simulink model "pvt_tegs_vienna"  (R2023b)
settings: Solver=ode14x  StartTime=0.0  StopTime=3*24*3600  FixedStep=1  RelTol=1e-06
PreLoadFcn:
  | sscv_hybrid_solar_panel_data
values from neighbouring files (symbols this model uses):
  Inclination = struct()    [meteo_data_struct.m]
  Irradiance_si = struct()    [meteo_data_struct.m]
  Irradiance_ts = struct()    [meteo_data_struct.m]
  load = struct()    [pvt_tegs_data.m]
  month = months{m}    [AUTOMATICO_mix.m]    (also in AUTOMATICO_parallel.m; AUTOMATICO_series.m)
  panel = struct()    [pvt_tegs_data.m]
  pipe = struct()    [pvt_tegs_data.m]
  pumps = struct()    [pvt_tegs_data.m]
  T_ext = struct()    [meteo_data_struct.m]
  tank = struct()    [pvt_tegs_data.m]
  teg = struct()    [pvt_tegs_data.m]
libraries: fl_lib x69, nesl_utility x35, simulink x5, ee_lib x2, My_second_lib x1, SimscapeFluids_lib x1
(part 1 of 2)
CloseFcn:
  | try,close(figHandleSolarInputs),end
  | clear figHandleSolarInputs
  | try,close(figHandlePumpInputs),end
  | clear figHandlePumpInputs
  | try,close(figHandleOptics),end
  | clear figHandleOptics
  | try,close(figHandleOutputs),end
  | clear figHandleOutputs
Description:
  | Photovoltaic Thermal Hybrid Solar Panel.
  | %
settings Model: Creator=The MathWorks, Inc.  LastModifiedBy=Utente
settings SolverCC: MaxConsecutiveMinStep=10  MaxZcPerStep=1
settings DataIOCC: SaveOutput=off  SignalLogging=off  DSMLogging=off
settings OptimizationCC: ReuseModelBlockBuffer=off
settings DebuggingCC: UnconnectedInputMsg=warning  UnconnectedOutputMsg=warning  UnconnectedLineMsg=warning  ArithmeticOperatorsInVariantConditions=warning
settings ModelReferenceCC: EnableRefExpFcnMdlSchedulingChecks=on
settings SFSimCC: SimUseLocalCustomCode=off
settings RTWCC: RTWUseLocalCustomCode=off  DLArmComputeVersion=19.05
settings SimscapeCC: SimscapeLogType=all  SimscapeLogSimulationStatistics=on  SimscapeLogName=simlog_hybrid_solar_panel  SimscapeLogDataHistory=10000

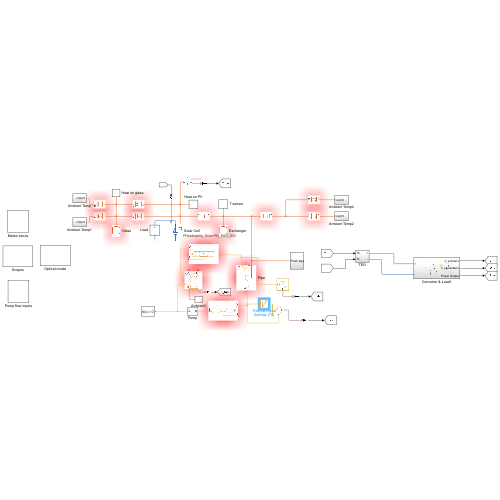
[thumbnail: Simulink's stored preview of the top-level diagram]
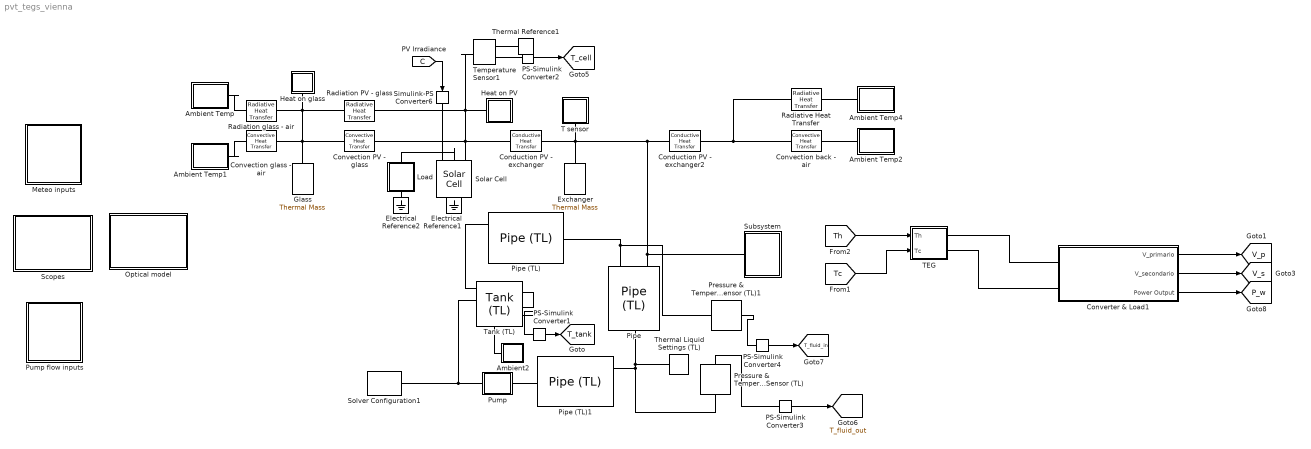
== system pvt_tegs_vienna ==
  Ambient Temp : Subsystem
  Ambient Temp1 : Subsystem
  Ambient Temp2 : Subsystem
  Ambient Temp4 : Subsystem
  Ambient2 : Subsystem
  Conduction PV - exchanger : fl_lib/Thermal/Thermal Elements/Conductive Heat Transfer  thermal_type=foundation.enum.ConstantVariableTabulated.Constant  wall_geometry=foundation.enum.ConductionWallGeometry.Planar  area=panel.geometry.Ncell*panel.geometry.Acell m^2  thickness=panel.heatTransfer.Le m  d_in=0.05 m  d_out=0.1 m  L=1 m  th_cond_min=10 W/(K*m)  th_cond=panel.heatTransfer.ke W/(m*K)  th_cond_TLU=[413, 401, 392, 383, 371, 357, 342] W/(K*m)  temp_TLU=[200, 273, 400, 600, 800, 1000, 1200] K  T_specify=off  T_priority=None  T=0 K  T_nominal_specify=off  T_nominal_unit=K  T_nominal_value=1  Q_specify=off  Q_priority=None  Q=0 W  Q_nominal_specify=off  Q_nominal_unit=W  Q_nominal_value=1
  Conduction PV - exchanger2 : fl_lib/Thermal/Thermal Elements/Conductive Heat Transfer  thermal_type=foundation.enum.ConstantVariableTabulated.Constant  wall_geometry=foundation.enum.ConductionWallGeometry.Planar  area=panel.geometry.Ncell*panel.geometry.Acell-teg.A_tot m^2  thickness=panel.heatTransfer.Le m  d_in=0.05 m  d_out=0.1 m  L=1 m  th_cond_min=10 W/(K*m)  th_cond=panel.heatTransfer.ke W/(m*K)  th_cond_TLU=[413, 401, 392, 383, 371, 357, 342] W/(K*m)  temp_TLU=[200, 273, 400, 600, 800, 1000, 1200] K  T_specify=off  T_priority=None  T=0 K  T_nominal_specify=off  T_nominal_unit=K  T_nominal_value=1  Q_specify=off  Q_priority=None  Q=0 W  Q_nominal_specify=off  Q_nominal_unit=W  Q_nominal_value=1
  Convection PV - glass : fl_lib/Thermal/Thermal Elements/Convective Heat Transfer  thermal_type=foundation.enum.constant_variable.constant  area=panel.geometry.Ncell*panel.geometry.Acell m^2  heat_tr_coeff=panel.heatTransfer.hgpv W/(m^2 * K)  min_heat_tr_coeff=1e-3 W/(K*m^2)  T_specify=off  T_priority=None  T=0 K  T_nominal_specify=off  T_nominal_unit=K  T_nominal_value=1  Q_specify=off  Q_priority=None  Q=0 W  Q_nominal_specify=off  Q_nominal_unit=W  Q_nominal_value=1
  Convection back - air : fl_lib/Thermal/Thermal Elements/Convective Heat Transfer  thermal_type=foundation.enum.constant_variable.constant  area=panel.geometry.Ncell*panel.geometry.Acell-teg.A_tot m^2  heat_tr_coeff=panel.heatTransfer.hba W/(m^2 * K)  min_heat_tr_coeff=1e-3 W/(K*m^2)  T_specify=off  T_priority=None  T=0 K  T_nominal_specify=off  T_nominal_unit=K  T_nominal_value=1  Q_specify=off  Q_priority=None  Q=0 W  Q_nominal_specify=off  Q_nominal_unit=W  Q_nominal_value=1
  Convection glass - air : fl_lib/Thermal/Thermal Elements/Convective Heat Transfer  thermal_type=foundation.enum.constant_variable.constant  area=panel.geometry.Ncell*panel.geometry.Acell m^2  heat_tr_coeff=panel.heatTransfer.hga W/(m^2 * K)  min_heat_tr_coeff=1e-3 W/(K*m^2)  T_specify=off  T_priority=None  T=0 K  T_nominal_specify=off  T_nominal_unit=K  T_nominal_value=1  Q_specify=off  Q_priority=None  Q=0 W  Q_nominal_specify=off  Q_nominal_unit=W  Q_nominal_value=1
  Converter & Load1 : Subsystem
  Electrical Reference1 : fl_lib/Electrical/Electrical Elements/Electrical Reference
  Electrical Reference2 : fl_lib/Electrical/Electrical Elements/Electrical Reference
  Exchanger : fl_lib/Thermal/Thermal Elements/Thermal Mass  mass_type=foundation.enum.constant_variable.constant  mass=panel.heatTransfer.Me kg  sp_heat=panel.heatTransfer.Ce J/kg/K  mass_min=1e-6 kg  num_ports=foundation.enum.numPorts2.one  m_specify=off  m_priority=High  m=1 kg  m_nominal_specify=off  m_nominal_unit=kg  m_nominal_value=1  T_specify=on  T_priority=High  T=panel.initial.Te0 K  T_nominal_specify=off  T_nominal_unit=K  T_nominal_value=1  Q_specify=off  Q_priority=None  Q=0 W  Q_nominal_specify=off  Q_nominal_unit=W  Q_nominal_value=1
  Glass : fl_lib/Thermal/Thermal Elements/Thermal Mass  mass_type=foundation.enum.constant_variable.constant  mass=panel.heatTransfer.Mg kg  sp_heat=panel.heatTransfer.Cg J/kg/K  mass_min=1e-6 kg  num_ports=foundation.enum.numPorts2.one  m_specify=off  m_priority=High  m=1 kg  m_nominal_specify=off  m_nominal_unit=kg  m_nominal_value=1  T_specify=on  T_priority=High  T=panel.initial.Tg0 K  T_nominal_specify=off  T_nominal_unit=K  T_nominal_value=1  Q_specify=off  Q_priority=None  Q=0 W  Q_nominal_specify=off  Q_nominal_unit=W  Q_nominal_value=1
  Heat on PV : Subsystem
  Heat on glass : Subsystem
  Load : Subsystem
  Meteo inputs : Subsystem
  Optical model : Subsystem
  PS-Simulink Converter1 : nesl_utility/PS-Simulink Converter  PhysicalDomain=network_engine_domain  SubClassName=ps_output  LeftPortType=input  RightPortType=output  PseudoPeriodic=off  Frequencies=[]  VectorFormat=inherit  Unit=inherit  AffineConversion=off
  PS-Simulink Converter2 : nesl_utility/PS-Simulink Converter  PhysicalDomain=network_engine_domain  SubClassName=ps_output  LeftPortType=input  RightPortType=output  PseudoPeriodic=off  Frequencies=[]  VectorFormat=inherit  Unit=K  AffineConversion=off
  PS-Simulink Converter3 : nesl_utility/PS-Simulink Converter  PhysicalDomain=network_engine_domain  SubClassName=ps_output  LeftPortType=input  RightPortType=output  PseudoPeriodic=off  Frequencies=[]  VectorFormat=inherit  Unit=inherit  AffineConversion=off
  PS-Simulink Converter4 : nesl_utility/PS-Simulink Converter  PhysicalDomain=network_engine_domain  SubClassName=ps_output  LeftPortType=input  RightPortType=output  PseudoPeriodic=off  Frequencies=[]  VectorFormat=inherit  Unit=inherit  AffineConversion=off
  Pipe : fl_lib/Thermal Liquid/Elements/Pipe (TL)  length=pipe.hx m  area=pipe.area m^2  Dh=pipe.Dh m  length_add=pipe.hx_eq_length m  roughness=pipe.roughness m  Re_lam=pipe.Re_lam  Re_tur=pipe.Re_tur  shape_factor=pipe.shape_factor  Nu_lam=pipe.Nu_lam  dynamic_compressibility=simscape.enum.onoff.off  inertia=simscape.enum.onoff.off  p0=0.101325 MPa  T0=Tm_month K  mdot0=0 kg/s
  Pipe (TL) : fl_lib/Thermal Liquid/Elements/Pipe (TL)  length=pipe.length m  area=pipe.area m^2  Dh=pipe.Dh m  length_add=pipe.eq_length1 m  roughness=pipe.roughness m  Re_lam=pipe.Re_lam  Re_tur=pipe.Re_tur  shape_factor=pipe.shape_factor  Nu_lam=pipe.Nu_lam  dynamic_compressibility=false  inertia=false  p0=0.101325 MPa  T0=Tm_month K  mdot0=0 kg/s
  Pipe (TL)1 : fl_lib/Thermal Liquid/Elements/Pipe (TL)  length=pipe.length m  area=pipe.area m^2  Dh=pipe.Dh m  length_add=pipe.eq_length2 m  roughness=pipe.roughness m  Re_lam=pipe.Re_lam  Re_tur=pipe.Re_tur  shape_factor=pipe.shape_factor  Nu_lam=pipe.Nu_lam  dynamic_compressibility=false  inertia=false  p0=0.101325 MPa  T0=Tm_month K  mdot0=0 kg/s
  Pressure & Temperature Sensor (TL) : fl_lib/Thermal Liquid/Sensors/Pressure & Temperature Sensor (TL)  reference=foundation.enum.MeasurementReference.absolute  pressure=false  pressure_spec=foundation.enum.PressureMeasementSpec.Absolute  temperature=true
      settings: InternalSimscapePortConfiguration="{\"Bottom\":[{\"id\":\"T\",\"label\":\"T\",\"type\":\"output\"}],\"Left\":[{\"id\":\"A\",\"label\":\"A\",\"type\":\"foundation.thermal_liquid.thermal_liquid\"}],\"Right\":[],\"Top\":[]}"
  Pressure & Temperature Sensor (TL)1 : fl_lib/Thermal Liquid/Sensors/Pressure & Temperature Sensor (TL)  reference=foundation.enum.MeasurementReference.absolute  pressure=false  pressure_spec=foundation.enum.PressureMeasementSpec.Absolute  temperature=true
      settings: InternalSimscapePortConfiguration="{\"Bottom\":[{\"id\":\"T\",\"label\":\"T\",\"type\":\"output\"}],\"Left\":[{\"id\":\"A\",\"label\":\"A\",\"type\":\"foundation.thermal_liquid.thermal_liquid\"}],\"Right\":[],\"Top\":[]}"
  Pump : Subsystem
  Pump flow inputs : Subsystem
  Radiation PV - glass : fl_lib/Thermal/Thermal Elements/Radiative Heat Transfer  area=panel.geometry.Ncell*panel.geometry.Acell m^2  rad_tr_coeff=5.670367e-8/(1/panel.heatTransfer.epsg + 1/panel.heatTransfer.epspv - 1) W/(m^2*K^4)  T_specify=off  T_priority=None  T=0 K  T_nominal_specify=off  T_nominal_unit=K  T_nominal_value=1  Q_specify=off  Q_priority=None  Q=0 W  Q_nominal_specify=off  Q_nominal_unit=W  Q_nominal_value=1
      settings: InternalSimscapePortConfiguration="{\"Bottom\":[],\"Left\":[{\"id\":\"A\",\"label\":\"A\",\"type\":\"foundation.thermal.thermal\"}],\"Right\":[{\"id\":\"B\",\"label\":\"B\",\"type\":\"foundation.thermal.thermal\"}],\"Top\":[]}"
  Radiation glass - air : fl_lib/Thermal/Thermal Elements/Radiative Heat Transfer  area=panel.geometry.Ncell*panel.geometry.Acell m^2  rad_tr_coeff=5.670367e-8*panel.heatTransfer.epsg W/(m^2*K^4)  T_specify=off  T_priority=None  T=0 K  T_nominal_specify=off  T_nominal_unit=K  T_nominal_value=1  Q_specify=off  Q_priority=None  Q=0 W  Q_nominal_specify=off  Q_nominal_unit=W  Q_nominal_value=1
      settings: InternalSimscapePortConfiguration="{\"Bottom\":[],\"Left\":[{\"id\":\"A\",\"label\":\"A\",\"type\":\"foundation.thermal.thermal\"}],\"Right\":[{\"id\":\"B\",\"label\":\"B\",\"type\":\"foundation.thermal.thermal\"}],\"Top\":[]}"
  Radiative Heat Transfer : fl_lib/Thermal/Thermal Elements/Radiative Heat Transfer  area=panel.geometry.Ncell*panel.geometry.Acell-teg.A_tot m^2  rad_tr_coeff=5.670367e-8/(1/pipe.emiss + 1/pipe.emiss_bricks - 1) W/(K^4*m^2)  T_specify=off  T_priority=None  T=0 K  T_nominal_specify=off  T_nominal_unit=K  T_nominal_value=1  Q_specify=off  Q_priority=None  Q=0 W  Q_nominal_specify=off  Q_nominal_unit=W  Q_nominal_value=1
      settings: InternalSimscapePortConfiguration="{\"Bottom\":[],\"Left\":[{\"id\":\"A\",\"label\":\"A\",\"type\":\"foundation.thermal.thermal\"}],\"Right\":[{\"id\":\"B\",\"label\":\"B\",\"type\":\"foundation.thermal.thermal\"}],\"Top\":[]}"
  Scopes : Subsystem
  Simulink-PS Converter6 : nesl_utility/Simulink-PS Converter  PhysicalDomain=network_engine_domain  SubClassName=ps_input  LeftPortType=input  RightPortType=output  PseudoPeriodic=off  Frequencies=[]  NoiseDistribution=none  NoiseParameters=[]  Unit=W/m^2  AffineConversion=off  FilteringAndDerivatives=provide  SimscapeFilterOrder=1  InputFilterTimeConstant=0.001  UdotUserProvided=0
  Solar Cell : ee_lib/Sources/Solar Cell  Tag={'toolbox/physmod/elec/library/m/ee_lib_parts';'Sources/Solar_Cell/Philadelphia_Solar/PS_M60_305.xml'}  prm=3  Isc=9.78 A  Voc=0.66918 V  Is=2.35776661208729e-07 A  Is2=1.71964843290271e-09 A  Iph=9.78001180187482 A  Ir0=1000 W/m^2  ec=1.48486924498379  N2=1.8278696613491  Rs=0.000864040468174528 Ohm  Rp=759.804445024526 Ohm  N_series=60  N_parallel=1  TIPH1=0.000600001676771431 1/K  EG=1.12 eV  TXIS1=5.6792037392937  TXIS2=14.7305501462979  TRS1=0.146242343009721  TRP1=0 % Parameter not set  Tmeas=25 degC  TFIXED=25 degC  thermal_mass=100 % Parameter not set J/K  initial_temperature=25 degC
      settings: AttributesFormatString=Philadelphia_Solar:PS_M60_305  InternalSimscapePortConfiguration="{\"Bottom\":[],\"Left\":[{\"id\":\"Ir\",\"label\":\"Ir\",\"type\":\"input\"},{\"id\":\"p\",\"label\":\"+\",\"type\":\"foundation.electrical.electrical\"},{\"id\":\"H\",\"label\":\"H\",\"type\":\"foundation.thermal.thermal\"}],\"Right\":[{\"id\":\"n\",\"label\":\"-\",\"type\":\"foundation.electrical.electrical\"}],\"Top\":[]}"
  Solver Configuration1 : nesl_utility/Solver Configuration  PhysicalDomain=network_engine_domain  SubClassName=solver  LeftPortType=input  RightPortType=generic  Tones=[]  Harmonics=[]  SimulateNoise=off  Profile=off  UseLocalSampling=off  EnableSwitchedLinearOptims=on  FrequencyDomain=off  UseCCode=off  RelTol=0.001  AbsTol=0.001  MinStep=1e-09  ToWorkspace=off  RevertToSquareIcSolve=off  NumHomotopyIterations=100  PhasorMode=off  PhasorModeNumHarmonics=1  ConsistencySolver=NEWTON_XTOL_AFTER_FTOL  IndexReductionMethod=DerivativeReplacement  DoDC=off  ResidualTolerance=1e-09  ConsistencyTolSource=GLOBAL  ConsistencyAbsTol=0.001  ConsistencyRelTol=0.001  ConsistencyTolFactor=0.001  UseLocalSolver=off  LocalSolverChoice=NE_BACKWARD_EULER_ADVANCER  ResolveIndetEquations=on  FunctionEvalNumThread=1  LocalSolverSampleTime=0.001  DoFixedCost=off  MaxNonlinIter=3  MaxModeIter=2  ComputeImpulses=off  ImpulseIterations=2  LinearAlgebra=auto  LinearAlgebraNumThread=0  EquationFormulation=NE_TIME_EF  DelaysMemoryBudget=1024  AutomaticFiltering=on  FilteringTimeConstant=0.001  PartitionStorageMethod=AS_NEEDED  PartitionMemoryBudget=1024  PartitionMethod=ROBUST  MultibodyUseLocalSolver=off  MultibodyLocalSolverChoice=ODE1  MultibodyLocalSolverSampleTime=0.001
  Subsystem : Subsystem
  T sensor : Subsystem
  TEG : Subsystem
  Tank (TL) : SimscapeFluids_lib/Thermal Liquid/Tanks & Accumulators/Tank (TL)  num_inlet=fluids.thermal_liquid.tanks_accumulators.enum.NumInlet.Two  pressure_spec=fluids.thermal_liquid.tanks_accumulators.enum.TankPressureSpec.Atmospheric  tank_pressure=0.101325 MPa  volume_spec=fluids.thermal_liquid.tanks_accumulators.enum.TankVolumeSpec.Constant  tank_area=tank.Atank m^2  level_TLU=[0, 3, 5] m  volume_TLU=[0, 4, 6] m^3  inlet_height_A=0.1 m  inlet_area_A=0.01 m^2  inlet_heights_AB=[0,0] m  inlet_areas_AB=[tank.Atank,tank.Atank] m^2  inlet_heights_ABC=[.1, .1, .1] m  inlet_areas_ABC=[.01, .01, .01] m^2  inlet_heights_ABCD=0.1 * ones(1, 4) m  inlet_areas_ABCD=0.01 * ones(1, 4) m^2  inlet_heights_ABCDE=0.1 * ones(1, 5) m  inlet_areas_ABCDE=0.01 * ones(1, 5) m^2  inlet_heights_ABCDEF=0.1 * ones(1, 6) m  inlet_areas_ABCDEF=0.01 * ones(1, 6) m^2  level_check=simscape.enum.assert.action.error  capacity_check=simscape.enum.assert.action.warn  max_capacity=tank.Volmax m^3  g=9.81 m/s^2  level_specify=on  level_priority=Low  level=tank.Voltank0/tank.Atank m  level_nominal_specify=off  level_nominal_unit=m  level_nominal_value=1  volume_specify=on  volume_priority=High  volume=tank.Voltank0 m^3  volume_nominal_specify=off  volume_nominal_unit=m^3  volume_nominal_value=1  mass_specify=off  mass_priority=None  mass=5000 kg  mass_nominal_specify=off  mass_nominal_unit=kg  mass_nominal_value=1  T_I_specify=on  T_I_priority=High  T_I=Tm_month K  T_I_nominal_specify=off  T_I_nominal_unit=K  T_I_nominal_value=1
      settings: InternalSimscapePortConfiguration="{\"Bottom\":[{\"id\":\"H\",\"label\":\"H\",\"type\":\"foundation.thermal.thermal\"},{\"id\":\"T_out\",\"label\":\"T\",\"type\":\"output\"}],\"Left\":[{\"id\":\"A\",\"label\":\"A\",\"type\":\"foundation.thermal_liquid.thermal_liquid\"},{\"id\":\"B\",\"label\":\"B\",\"type\":\"foundation.thermal_liquid.thermal_liquid\"}],\"Right\":[],\"Top\":[{\"id\":\"V_out\",\"label\":\"V\",\"type\":\"output\"},{\"id\":\"L_out\",\"label\":\"L\",\"type\":\"output\"}]}"
  Temperature Sensor1 : fl_lib/Thermal/Thermal Sensors/Temperature Sensor  temperature_measure=foundation.enum.MeasurementReference.difference
  Thermal Liquid Settings (TL) : fl_lib/Thermal Liquid/Utilities/Thermal Liquid Settings (TL)  table_dimensions=foundation.enum.table_dimensions_TL.one_dimensional  T_TLU=[263.16, 273.16:20:373.16]' K  p_TLU=[0.01, 0.1, 5 : 5 : 50] MPa  p_atm=0.101325 MPa  pT_region_flag=foundation.enum.pT_region_TL.min_max  T_min=273.16 K  T_max=363.16 K  p_min=0.05 MPa  p_max=50 MPa  T_min_1D=263.16 K  T_max_1D=373.16 K  p_min_1D=0.05 MPa  p_max_1D=50 MPa  pT_validity_TLU=[1, 1, 1, 1, 1, 1, 1, 1, 1, 1, 1, 1; 1, 1, 1, 1, 1, 1, 1, 1, 1, 1, 1, 1; 1, 1, 1, 1, 1, 1, 1, 1, 1, 1, 1, 1; 1, 1, 1, 1, 1, 1, 1, 1, 1, 1, 1, 1; 1, 1, 1, 1, 1, 1, 1, 1, 1, 1, 1, 1; 0, 1, 1, 1, 1, 1, 1, 1, 1, 1, 1, 1; 0, 1, 1, 1, 1, 1, 1, 1, 1, 1, 1, 1; 0, 1, 1, 1, 1, 1, 1, 1, 1, 1, 1, 1; 0, 1, 1, 1, 1, 1, 1, 1, 1, 1, 1, 1; 0, 1, 1, 1, 1, 1, 1, 1, 1, 1, 1, 1; 0, 0, 1, 1, 1, 1, 1, 1, 1, 1, 1, 1]  properties_range_check=simscape.enum.assert.action.error  rho_parameterization_2D=foundation.enum.rho_parameterization_2D.rho_beta_alpha  rho_parameterization_1D=foundation.enum.rho_parameterization_1D.rho_vector  rho_TLU=[999.7973, 999.8431, 1002.3216, 1004.8218, 1007.293, 1009.7358, 1012.1506, 1014.5379, 1016.8979, 1019.2311, 1021.538, 1023.8188; 999.6579, 999.7009, 1002.0303, 1004.382, 1006.7084, 1009.0101, 1011.2874, 1013.5407, 1015.7703, 1017.9766, 1020.1599, 1022.3206; 998.1632, 998.2045, 1000.4375, 1002.6924, 1004.9239, 1007.1324, 1009.3183, 1011.4819, 1013.6236, 1015.7438, 1017.8428, 1019.921; 995.6057, 995.6458, 997.81864, 1000.0128, 1002.1841, 1004.3332, 1006.4603, 1008.566, 1010.6505, 1012.7144, 1014.758, 1016.7815; 992.1724, 992.2119, 994.35133, 996.5113, 998.6484, 1000.7633, 1002.8563, 1004.928, 1006.9788, 1009.009, 1011.0192, 1013.0097; 988.02, 988.0299, 990.15684, 992.3035, 994.4268, 996.5273, 998.6056, 1000.6622, 1002.6976, 1004.7123, 1006.7067, 1008.6813; 983.18, 983.1901, 985.3217, 987.4721, 989.5983, 991.7008, 993.7803, 995.8374, 997.8726, 999.8864, 1001.8795, 1003.8522; 977.75, 977.7583, 979.9094, 982.0783, 984.2216, 986.34, 988.4343, 990.505, 992.5529, 994.5786, 996.5825, 998.5654; 971.77, 971.7836, 973.96734, 976.1678, 978.3409, 980.4876, 982.6087, 984.7049, 986.7768, 988.8254, 990.8511, 992.8545; 965.26, 965.3023, 967.53107, 969.7753, 971.9901, 974.1764, 976.3354, 978.4676, 980.5741, 982.6556, 984.7129, 986.7465; 958.62, 958.6315, 960.627, 962.9267, 965.1944, 967.4314, 969.6387, 971.8173, 973.9681, 976.0921, 978.19, 980.2628] kg/m^3  beta_TLU=[1.9649, 1.9654, 1.9929, 2.0213, 2.0499, 2.0787, 2.1078, 2.1372, 2.1668, 2.1966, 2.2268, 2.2572; 2.0913, 2.0918, 2.1191, 2.1471, 2.1752, 2.2036, 2.2322, 2.261, 2.2899, 2.3191, 2.3485, 2.3781; 2.1786, 2.1791, 2.2067, 2.235, 2.2634, 2.2919, 2.3206, 2.3494, 2.3784, 2.4075, 2.4367, 2.4661; 2.2332, 2.2337, 2.2619, 2.2908, 2.3197, 2.3487, 2.3778, 2.407, 2.4363, 2.4657, 2.4951, 2.5246; 2.26, 2.2605, 2.2895, 2.3191, 2.3487, 2.3784, 2.4081, 2.4378, 2.4675, 2.4973, 2.5272, 2.5571; 2.2638, 2.2638, 2.2936, 2.324, 2.3544, 2.3848, 2.4151, 2.4455, 2.4758, 2.5062, 2.5365, 2.5669; 2.2472, 2.2472, 2.2779, 2.3092, 2.3403, 2.3715, 2.4025, 2.4336, 2.4646, 2.4955, 2.5264, 2.5573; 2.214, 2.214, 2.2455, 2.2776, 2.3096, 2.3415, 2.3733, 2.405, 2.4367, 2.4683, 2.4998, 2.5313; 2.1668, 2.1668, 2.1992, 2.2321, 2.2649, 2.2976, 2.3301, 2.3626, 2.3949, 2.4272, 2.4593, 2.4914; 2.1081, 2.1081, 2.1413, 2.175, 2.2086, 2.2421, 2.2754, 2.3085, 2.3415, 2.3744, 2.4072, 2.4399; 2.0494, 2.0494, 2.0739, 2.1084, 2.1428, 2.177, 2.211, 2.2449, 2.2786, 2.3121, 2.3455, 2.3788] GPa  alpha_TLU=1e-4 * [-.679, -.676, -.49, -.307, -.13, .041, .206, .365, .519, .668, .811, .949; .878, .881, .998, 1.114, 1.227, 1.337, 1.445, 1.549, 1.651, 1.75, 1.846, 1.939; 2.068, 2.069, 2.141, 2.213, 2.283, 2.352, 2.42, 2.486, 2.551, 2.614, 2.676, 2.736; 3.034, 3.035, 3.074, 3.113, 3.152, 3.191, 3.229, 3.267, 3.305, 3.341, 3.377, 3.413; 3.855, 3.856, 3.87, 3.884, 3.899, 3.914, 3.93, 3.946, 3.961, 3.977, 3.993, 4.009; 4.578, 4.578, 4.572, 4.566, 4.562, 4.558, 4.555, 4.552, 4.55, 4.549, 4.548, 4.547; 5.233, 5.233, 5.209, 5.186, 5.165, 5.144, 5.125, 5.107, 5.09, 5.074, 5.059, 5.045; 5.84, 5.84, 5.801, 5.762, 5.725, 5.691, 5.657, 5.625, 5.595, 5.566, 5.538, 5.512; 6.414, 6.414, 6.36, 6.307, 6.256, 6.208, 6.161, 6.117, 6.074, 6.033, 5.994, 5.956; 6.967, 6.967, 6.898, 6.831, 6.766, 6.705, 6.646, 6.589, 6.535, 6.482, 6.432, 6.384; 7.519, 7.519, 7.423, 7.342, 7.264, 7.189, 7.118, 7.049, 6.983, 6.92, 6.859, 6.8] 1/K  rho_TLU_2=[999.7973, 999.8431, 1002.3216, 1004.8218, 1007.293, 1009.7358, 1012.1506, 1014.5379, 1016.8979, 1019.2311, 1021.538, 1023.8188; 999.6579, 999.7009, 1002.0303, 1004.382, 1006.7084, 1009.0101, 1011.2874, 1013.5407, 1015.7703, 1017.9766, 1020.1599, 1022.3206; 998.1632, 998.2045, 1000.4375, 1002.6924, 1004.9239, 1007.1324, 1009.3183, 1011.4819, 1013.6236, 1015.7438, 1017.8428, 1019.921; 995.6057, 995.6458, 997.81864, 1000.0128, 1002.1841, 1004.3332, 1006.4603, 1008.566, 1010.6505, 1012.7144, 1014.758, 1016.7815; 992.1724, 992.2119, 994.35133, 996.5113, 998.6484, 1000.7633, 1002.8563, 1004.928, 1006.9788, 1009.009, 1011.0192, 1013.0097; 988.02, 988.0299, 990.15684, 992.3035, 994.4268, 996.5273, 998.6056, 1000.6622, 1002.6976, 1004.7123, 1006.7067, 1008.6813; 983.18, 983.1901, 985.3217, 987.4721, 989.5983, 991.7008, 993.7803, 995.8374, 997.8726, 999.8864, 1001.8795, 1003.8522; 977.75, 977.7583, 979.9094, 982.0783, 984.2216, 986.34, 988.4343, 990.505, 992.5529, 994.5786, 996.5825, 998.5654; 971.77, 971.7836, 973.96734, 976.1678, 978.3409, 980.4876, 982.6087, 984.7049, 986.7768, 988.8254, 990.8511, 992.8545; 965.26, 965.3023, 967.53107, 969.7753, 971.9901, 974.1764, 976.3354, 978.4676, 980.5741, 982.6556, 984.7129, 986.7465; 958.62, 958.6315, 960.627, 962.9267, 965.1944, 967.4314, 969.6387, 971.8173, 973.9681, 976.0921, 978.19, 980.2628] kg/m^3  rho_ref_3=998.21 kg/m^3  T_ref_3=293.16 K  p_ref_3=0.101325 MPa  beta_const_3=2.1791 GPa  alpha_const_3=2.0691e-4 1/K  rho_TLU_4=[1038, 1036, 1030, 1022, 1014, 1006, 997]' kg/m^3  beta_const_4=3.4 GPa  p_ref_4=0.101325 MPa  rho_ref_5=998.21 kg/m^3  T_ref_5=293.16 K  p_ref_5=0.101325 MPa  beta_const_5=2.1791 GPa  alpha_const_5=2.0691e-4 1/K  u_parameterization_2D=foundation.enum.u_parameterization_2D.u_cp  u_parameterization_1D=foundation.enum.u_parameterization_1D.cp  u_TLU=[.0002, .0018, .086, .1588, .219, .267, .3034, .3288, .3436, .3483, .3435, .3294; 42.062, 42.06, 41.935, 41.804, 41.668, 41.527, 41.382, 41.233, 41.081, 40.924, 40.763, 40.599; 83.953, 83.948, 83.651, 83.349, 83.049, 82.749, 82.451, 82.153, 81.856, 81.56, 81.265, 80.971; 125.77, 125.76, 125.31, 124.86, 124.41, 123.97, 123.53, 123.1, 122.68, 122.25, 121.84, 121.42; 167.57, 167.56, 166.96, 166.37, 165.79, 165.21, 164.65, 164.09, 163.54, 163, 162.46, 161.94; 209.36, 209.36, 208.63, 207.9, 207.19, 206.48, 205.79, 205.11, 204.45, 203.79, 203.14, 202.5; 251.19, 251.19, 250.33, 249.47, 248.62, 247.79, 246.98, 246.18, 245.39, 244.62, 243.86, 243.12; 293.06, 293.06, 292.07, 291.07, 290.1, 289.14, 288.2, 287.28, 286.38, 285.49, 284.62, 283.77; 334.99, 334.99, 333.86, 332.73, 331.63, 330.54, 329.48, 328.44, 327.41, 326.41, 325.43, 324.46; 377, 377, 375.73, 374.46, 373.22, 372, 370.81, 369.64, 368.5, 367.38, 366.27, 365.19; 419.01, 419.01, 417.69, 416.27, 414.89, 413.54, 412.21, 410.91, 409.64, 408.4, 407.17, 405.98] kJ/kg  cp_TLU=[4.2199, 4.2194, 4.1957, 4.1726, 4.1508, 4.13, 4.1103, 4.0916, 4.0738, 4.0569, 4.0408, 4.0254; 4.1955, 4.1951, 4.1769, 4.1592, 4.1422, 4.1259, 4.1103, 4.0954, 4.0812, 4.0676, 4.0545, 4.0421; 4.1843, 4.184, 4.169, 4.1543, 4.1401, 4.1264, 4.1133, 4.1007, 4.0885, 4.0768, 4.0656, 4.0548; 4.1801, 4.1798, 4.1667, 4.1538, 4.1413, 4.1293, 4.1177, 4.1064, 4.0956, 4.0851, 4.075, 4.0653; 4.1796, 4.1794, 4.1675, 4.1558, 4.1444, 4.1334, 4.1227, 4.1123, 4.1023, 4.0926, 4.0832, 4.0741; 4.1813, 4.1813, 4.1702, 4.1592, 4.1484, 4.138, 4.1279, 4.1181, 4.1086, 4.0993, 4.0903, 4.0816; 4.185, 4.185, 4.1742, 4.1636, 4.1532, 4.1432, 4.1334, 4.1239, 4.1146, 4.1056, 4.0969, 4.0884; 4.1901, 4.1901, 4.1795, 4.169, 4.1588, 4.1489, 4.1393, 4.1299, 4.1207, 4.1118, 4.1032, 4.0947; 4.1968, 4.1968, 4.1862, 4.1757, 4.1655, 4.1555, 4.1458, 4.1364, 4.1273, 4.1183, 4.1096, 4.1012; 4.2052, 4.2052, 4.1944, 4.1837, 4.1733, 4.1632, 4.1534, 4.1438, 4.1345, 4.1255, 4.1166, 4.108; 4.2136, 4.2136, 4.2045, 4.1935, 4.1828, 4.1724, 4.1623, 4.1524, 4.1429, 4.1335, 4.1245, 4.1157] kJ/kg/K  u_TLU_2=[.0002, .0018, .086, .1588, .219, .267, .3034, .3288, .3436, .3483, .3435, .3294; 42.062, 42.06, 41.935, 41.804, 41.668, 41.527, 41.382, 41.233, 41.081, 40.924, 40.763, 40.599; 83.953, 83.948, 83.651, 83.349, 83.049, 82.749, 82.451, 82.153, 81.856, 81.56, 81.265, 80.971; 125.77, 125.76, 125.31, 124.86, 124.41, 123.97, 123.53, 123.1, 122.68, 122.25, 121.84, 121.42; 167.57, 167.56, 166.96, 166.37, 165.79, 165.21, 164.65, 164.09, 163.54, 163, 162.46, 161.94; 209.36, 209.36, 208.63, 207.9, 207.19, 206.48, 205.79, 205.11, 204.45, 203.79, 203.14, 202.5; 251.19, 251.19, 250.33, 249.47, 248.62, 247.79, 246.98, 246.18, 245.39, 244.62, 243.86, 243.12; 293.06, 293.06, 292.07, 291.07, 290.1, 289.14, 288.2, 287.28, 286.38, 285.49, 284.62, 283.77; 334.99, 334.99, 333.86, 332.73, 331.63, 330.54, 329.48, 328.44, 327.41, 326.41, 325.43, 324.46; 377, 377, 375.73, 374.46, 373.22, 372, 370.81, 369.64, 368.5, 367.38, 366.27, 365.19; 419.01, 419.01, 417.69, 416.27, 414.89, 413.54, 412.21, 410.91, 409.64, 408.4, 407.17, 405.98] kJ/kg  cp_TLU_3=[4.2199, 4.2194, 4.1957, 4.1726, 4.1508, 4.13, 4.1103, 4.0916, 4.0738, 4.0569, 4.0408, 4.0254; 4.1955, 4.1951, 4.1769, 4.1592, 4.1422, 4.1259, 4.1103, 4.0954, 4.0812, 4.0676, 4.0545, 4.0421; 4.1843, 4.184, 4.169, 4.1543, 4.1401, 4.1264, 4.1133, 4.1007, 4.0885, 4.0768, 4.0656, 4.0548; 4.1801, 4.1798, 4.1667, 4.1538, 4.1413, 4.1293, 4.1177, 4.1064, 4.0956, 4.0851, 4.075, 4.0653; 4.1796, 4.1794, 4.1675, 4.1558, 4.1444, 4.1334, 4.1227, 4.1123, 4.1023, 4.0926, 4.0832, 4.0741; 4.1813, 4.1813, 4.1702, 4.1592, 4.1484, 4.138, 4.1279, 4.1181, 4.1086, 4.0993, 4.0903, 4.0816; 4.185, 4.185, 4.1742, 4.1636, 4.1532, 4.1432, 4.1334, 4.1239, 4.1146, 4.1056, 4.0969, 4.0884; 4.1901, 4.1901, 4.1795, 4.169, 4.1588, 4.1489, 4.1393, 4.1299, 4.1207, 4.1118, 4.1032, 4.0947; 4.1968, 4.1968, 4.1862, 4.1757, 4.1655, 4.1555, 4.1458, 4.1364, 4.1273, 4.1183, 4.1096, 4.1012; 4.2052, 4.2052, 4.1944, 4.1837, 4.1733, 4.1632, 4.1534, 4.1438, 4.1345, 4.1255, 4.1166, 4.108; 4.2136, 4.2136, 4.2045, 4.1935, 4.1828, 4.1724, 4.1623, 4.1524, 4.1429, 4.1335, 4.1245, 4.1157] kJ/kg/K  u_TLU_4=[.0018; 42.06; 83.948; 125.76; 167.56; 209.36; 251.19; 293.06; 334.99; 377; 418.01] kJ/kg  cp_TLU_5=[3.85, 3.87, 3.90, 3.93, 3.96, 3.99, 4.02]' kJ/kg/K  nu_TLU=[1.7917, 1.7914, 1.7763, 1.7615, 1.7473, 1.7338, 1.7208, 1.7085, 1.6967, 1.6854, 1.6747, 1.6645; 1.3061, 1.3059, 1.2986, 1.2914, 1.2845, 1.2779, 1.2716, 1.2656, 1.2598, 1.2543, 1.2491, 1.2441; 1.0032, 1.0032, .9995, .9959, .9924, .9891, .9859, .9829, .9801, .9774, .9748, .9724; .8006, .8005, .7987, .797, .7953, .7937, .7922, .7908, .7894, .7881, .787, .7859; .6577, .6577, .657, .6562, .6555, .6548, .6543, .6537, .6532, .6528, .6523, .652; .553, .553, .5529, .5527, .5526, .5525, .5524, .5524, .5524, .5524, .5524, .5525; .4739, .4739, .4741, .4743, .4745, .4747, .475, .4753, .4755, .4758, .4762, .4765; .4127, .4127, .4131, .4135, .4139, .4143, .4148, .4152, .4157, .4162, .4167, .4172; .3643, .3643, .3648, .3654, .3659, .3665, .367, .3676, .3682, .3688, .3694, .37; .3254, .3254, .3261, .3267, .3273, .328, .3286, .3293, .3299, .3306, .3312, .3319; .2866, .2866, .2945, .2952, .2959, .2965, .2972, .2979, .2986, .2993, .3, .3007] mm^2/s  nu_TLU_2=[5, 3, 1.6, 1.0, 0.7, 0.52, 0.41]' mm^2/s  k_TLU=[561.04, 561.09, 563.8, 566.56, 569.32, 572.08, 574.82, 577.54, 580.24, 582.92, 585.57, 588.18; 580.02, 580.07, 582.45, 584.88, 587.32, 589.75, 592.18, 594.61, 597.02, 599.42, 601.8, 604.16; 598.44, 598.48, 600.73, 603.03, 605.33, 607.64, 609.94, 612.24, 614.54, 616.82, 619.1, 621.36; 615.48, 615.52, 617.73, 620, 622.26, 624.54, 626.81, 629.07, 631.34, 633.6, 635.85, 638.09; 630.6, 630.64, 632.87, 635.15, 637.44, 639.72, 642.01, 644.29, 646.57, 648.84, 651.11, 653.36; 643.61, 643.61, 645.88, 648.21, 650.53, 652.86, 655.18, 657.51, 659.82, 662.14, 664.44, 666.74; 654.39, 654.39, 656.73, 659.12, 661.5, 663.89, 666.27, 668.65, 671.02, 673.38, 675.74, 678.09; 663.13, 663.13, 665.54, 668, 670.46, 672.91, 675.36, 677.8, 680.24, 682.67, 685.09, 687.5; 670.02, 670.02, 672.51, 675.05, 677.59, 680.12, 682.64, 685.16, 687.67, 690.17, 692.66, 695.14; 675.27, 675.27, 677.85, 680.48, 683.11, 685.73, 688.34, 690.94, 693.53, 696.11, 698.68, 701.24; 680.52, 680.52, 681.77, 684.5, 687.22, 689.94, 692.64, 695.34, 698.02, 700.69, 703.35, 706] mW/m/K  k_TLU_2=[498, 500, 512, 521, 531, 540, 550]' mW/m/K
  Thermal Reference1 : fl_lib/Thermal/Thermal Elements/Thermal Reference
  tag scope: P_w=global, T_cell=global, T_fluid_in=global, T_fluid_out=global, T_tank=global, V_p=global, V_s=global
  wires:
  Converter & Load1/1(V_primario) -> [V_p]
  PS-Simulink Converter4/1 -> [T_fluid_in]
  Converter & Load1/3(Power Output) -> [P_w]
  Converter & Load1/2(V_secondario) -> [V_s]
  PS-Simulink Converter2/1 -> [T_cell]
  PS-Simulink Converter3/1 -> [T_fluid_out]
  [Tc] -> TEG/2(Tc)
  [C] -> Simulink-PS Converter6/1
  PS-Simulink Converter1/1 -> [T_tank]
  [Th] -> TEG/1(Th)
  connections:
  Pipe/LConn2 -- Subsystem/RConn1 -- Conduction PV - exchanger2/LConn1 -- Conduction PV - exchanger/RConn1 -- T sensor/LConn1 -- Exchanger/LConn1
  Pipe/RConn1 -- Thermal Liquid Settings (TL)/RConn1 -- Pressure & Temperature Sensor (TL)/LConn1 -- Pipe (TL)1/LConn1
  Pump/LConn1 -- Tank (TL)/LConn2 -- Solver Configuration1/RConn1
  Pipe/LConn1 -- Pipe (TL)/RConn1 -- Pressure & Temperature Sensor (TL)1/LConn1
  Radiation glass - air/LConn1 -- Convection glass - air/LConn1 -- Convection PV - glass/RConn1 -- Glass/LConn1 -- Radiation PV - glass/RConn1 -- Heat on glass/LConn1
  Convection back - air/LConn1 -- Radiative Heat Transfer/LConn1 -- Conduction PV - exchanger2/RConn1
  Convection PV - glass/LConn1 -- Radiation PV - glass/LConn1 -- Temperature Sensor1/LConn1 -- Heat on PV/LConn1 -- Conduction PV - exchanger/LConn1 -- Solar Cell/LConn3
  Thermal Reference1/LConn1 -- Temperature Sensor1/RConn1
  TEG/RConn2 -- Converter & Load1/LConn2
  Pressure & Temperature Sensor (TL)1/RConn1 -- PS-Simulink Converter4/LConn1
  Convection back - air/RConn1 -- Ambient Temp2/LConn1
  Temperature Sensor1/RConn2 -- PS-Simulink Converter2/LConn1
  Pipe (TL)1/RConn1 -- Pump/RConn1
  Solar Cell/RConn1 -- Electrical Reference1/LConn1
  PS-Simulink Converter3/LConn1 -- Pressure & Temperature Sensor (TL)/RConn1
  Ambient Temp4/LConn1 -- Radiative Heat Transfer/RConn1
  Ambient Temp/LConn1 -- Radiation glass - air/RConn1
  Solar Cell/LConn1 -- Simulink-PS Converter6/RConn1
  TEG/RConn1 -- Converter & Load1/LConn1
  Tank (TL)/RConn1 -- Ambient2/LConn1
  Ambient Temp1/LConn1 -- Convection glass - air/RConn1
  Tank (TL)/RConn2 -- PS-Simulink Converter1/LConn1
  Load/LConn1 -- Electrical Reference2/LConn1
  Pipe (TL)/LConn1 -- Tank (TL)/LConn1
  Solar Cell/LConn2 -- Load/RConn1

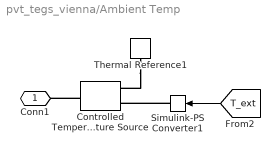
== system pvt_tegs_vienna/Ambient Temp ==
  Controlled Temperature Source : fl_lib/Thermal/Thermal Sources/Controlled Temperature Source
  Simulink-PS Converter1 : nesl_utility/Simulink-PS Converter  PhysicalDomain=network_engine_domain  SubClassName=ps_input  LeftPortType=input  RightPortType=output  PseudoPeriodic=off  Frequencies=[]  NoiseDistribution=none  NoiseParameters=[]  Unit=K  AffineConversion=off  FilteringAndDerivatives=provide  SimscapeFilterOrder=1  InputFilterTimeConstant=0.001  UdotUserProvided=0
  Thermal Reference1 : fl_lib/Thermal/Thermal Elements/Thermal Reference
  Conn1 : PMIOPort  Side=Left
  wires:
  [T_ext] -> Simulink-PS Converter1/1
  connections:
  Simulink-PS Converter1/RConn1 -- Controlled Temperature Source/RConn1
  Thermal Reference1/LConn1 -- Controlled Temperature Source/RConn2
  Controlled Temperature Source/LConn1 -- Conn1/RConn1

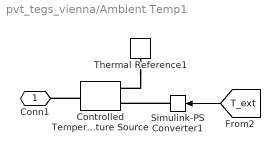
== system pvt_tegs_vienna/Ambient Temp1 ==
  Controlled Temperature Source : fl_lib/Thermal/Thermal Sources/Controlled Temperature Source
  Simulink-PS Converter1 : nesl_utility/Simulink-PS Converter  PhysicalDomain=network_engine_domain  SubClassName=ps_input  LeftPortType=input  RightPortType=output  PseudoPeriodic=off  Frequencies=[]  NoiseDistribution=none  NoiseParameters=[]  Unit=K  AffineConversion=off  FilteringAndDerivatives=provide  SimscapeFilterOrder=1  InputFilterTimeConstant=0.001  UdotUserProvided=0
  Thermal Reference1 : fl_lib/Thermal/Thermal Elements/Thermal Reference
  Conn1 : PMIOPort  Side=Left
  wires:
  [T_ext] -> Simulink-PS Converter1/1
  connections:
  Controlled Temperature Source/LConn1 -- Conn1/RConn1
  Thermal Reference1/LConn1 -- Controlled Temperature Source/RConn2
  Simulink-PS Converter1/RConn1 -- Controlled Temperature Source/RConn1

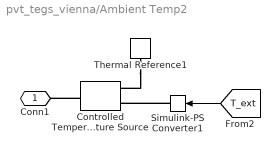
== system pvt_tegs_vienna/Ambient Temp2 ==
  Controlled Temperature Source : fl_lib/Thermal/Thermal Sources/Controlled Temperature Source
  Simulink-PS Converter1 : nesl_utility/Simulink-PS Converter  PhysicalDomain=network_engine_domain  SubClassName=ps_input  LeftPortType=input  RightPortType=output  PseudoPeriodic=off  Frequencies=[]  NoiseDistribution=none  NoiseParameters=[]  Unit=K  AffineConversion=off  FilteringAndDerivatives=provide  SimscapeFilterOrder=1  InputFilterTimeConstant=0.001  UdotUserProvided=0
  Thermal Reference1 : fl_lib/Thermal/Thermal Elements/Thermal Reference
  Conn1 : PMIOPort  Side=Left
  wires:
  [T_ext] -> Simulink-PS Converter1/1
  connections:
  Simulink-PS Converter1/RConn1 -- Controlled Temperature Source/RConn1
  Thermal Reference1/LConn1 -- Controlled Temperature Source/RConn2
  Controlled Temperature Source/LConn1 -- Conn1/RConn1

== system pvt_tegs_vienna/Ambient Temp4 ==
  Controlled Temperature Source : fl_lib/Thermal/Thermal Sources/Controlled Temperature Source
  Simulink-PS Converter1 : nesl_utility/Simulink-PS Converter  PhysicalDomain=network_engine_domain  SubClassName=ps_input  LeftPortType=input  RightPortType=output  PseudoPeriodic=off  Frequencies=[]  NoiseDistribution=none  NoiseParameters=[]  Unit=K  AffineConversion=off  FilteringAndDerivatives=provide  SimscapeFilterOrder=1  InputFilterTimeConstant=0.001  UdotUserProvided=0
  Thermal Reference1 : fl_lib/Thermal/Thermal Elements/Thermal Reference
  Conn1 : PMIOPort  Side=Left
  wires:
  [T_ext] -> Simulink-PS Converter1/1
  connections:
  Controlled Temperature Source/LConn1 -- Conn1/RConn1
  Thermal Reference1/LConn1 -- Controlled Temperature Source/RConn2
  Simulink-PS Converter1/RConn1 -- Controlled Temperature Source/RConn1

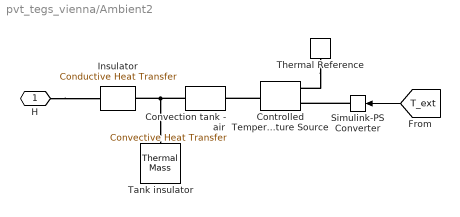
== system pvt_tegs_vienna/Ambient2 ==
  Controlled Temperature Source : fl_lib/Thermal/Thermal Sources/Controlled Temperature Source
  Convection tank - air : fl_lib/Thermal/Thermal Elements/Convective Heat Transfer  thermal_type=foundation.enum.constant_variable.constant  area=2*pi*sqrt(tank.Atank/pi)*tank.Volmax/tank.Atank+2*tank.Atank m^2  heat_tr_coeff=tank.hta W/(m^2 * K)  min_heat_tr_coeff=1e-3 W/(K*m^2)  T_specify=off  T_priority=None  T=0 K  T_nominal_specify=off  T_nominal_unit=K  T_nominal_value=1  Q_specify=off  Q_priority=None  Q=0 W  Q_nominal_specify=off  Q_nominal_unit=W  Q_nominal_value=1
  Insulator : fl_lib/Thermal/Thermal Elements/Conductive Heat Transfer  thermal_type=foundation.enum.ConstantVariableTabulated.Constant  wall_geometry=foundation.enum.ConductionWallGeometry.Planar  area=2*pi*sqrt(tank.Atank/pi)*tank.Volmax/tank.Atank+2*tank.Atank m^2  thickness=tank.Lins m  d_in=0.05 m  d_out=0.1 m  L=1 m  th_cond_min=10 W/(K*m)  th_cond=tank.kins W/(m*K)  th_cond_TLU=[413, 401, 392, 383, 371, 357, 342] W/(K*m)  temp_TLU=[200, 273, 400, 600, 800, 1000, 1200] K  T_specify=off  T_priority=None  T=0 K  T_nominal_specify=off  T_nominal_unit=K  T_nominal_value=1  Q_specify=off  Q_priority=None  Q=0 W  Q_nominal_specify=off  Q_nominal_unit=W  Q_nominal_value=1
  Simulink-PS Converter : nesl_utility/Simulink-PS Converter  PhysicalDomain=network_engine_domain  SubClassName=ps_input  LeftPortType=input  RightPortType=output  PseudoPeriodic=off  Frequencies=[]  NoiseDistribution=none  NoiseParameters=[]  Unit=K  AffineConversion=off  FilteringAndDerivatives=provide  SimscapeFilterOrder=1  InputFilterTimeConstant=0.001  UdotUserProvided=0
  Tank insulator : fl_lib/Thermal/Thermal Elements/Thermal Mass  mass_type=foundation.enum.constant_variable.constant  mass=tank.insul_mass kg  sp_heat=tank.spec_heat J/(K*kg)  mass_min=1e-6 kg  num_ports=foundation.enum.numPorts2.one  m_specify=off  m_priority=High  m=1 kg  m_nominal_specify=off  m_nominal_unit=kg  m_nominal_value=1  T_specify=off  T_priority=High  T=300 K  T_nominal_specify=off  T_nominal_unit=K  T_nominal_value=1  Q_specify=off  Q_priority=None  Q=0 W  Q_nominal_specify=off  Q_nominal_unit=W  Q_nominal_value=1
  Thermal Reference : fl_lib/Thermal/Thermal Elements/Thermal Reference
  H : PMIOPort  Side=Left
  wires:
  [T_ext] -> Simulink-PS Converter/1
  connections:
  H/RConn1 -- Insulator/LConn1
  Convection tank - air/LConn1 -- Insulator/RConn1 -- Tank insulator/LConn1
  Controlled Temperature Source/LConn1 -- Convection tank - air/RConn1
  Simulink-PS Converter/RConn1 -- Controlled Temperature Source/RConn1
  Thermal Reference/LConn1 -- Controlled Temperature Source/RConn2

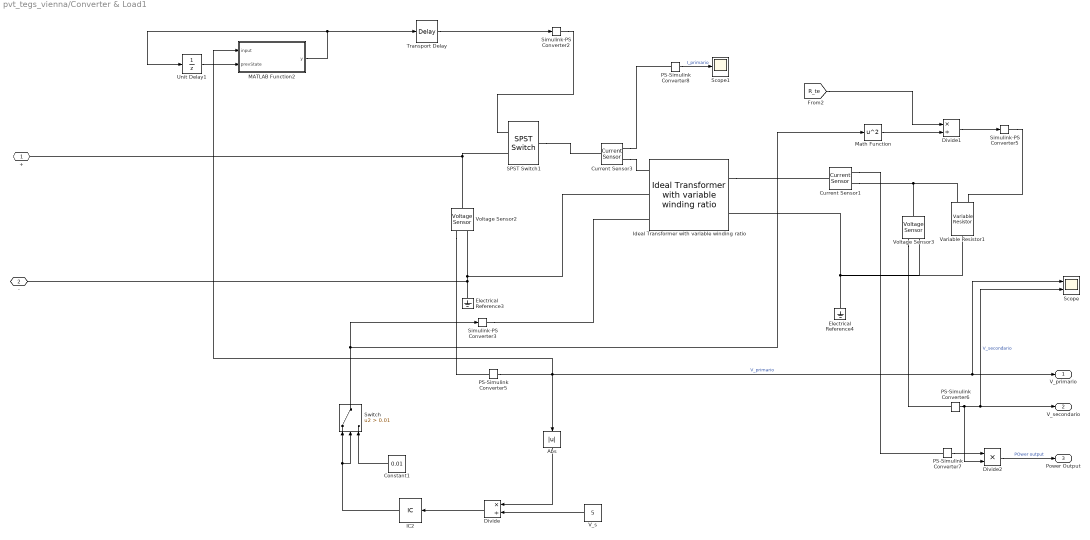
== system pvt_tegs_vienna/Converter & Load1 ==
  Abs : Abs  SaturateOnIntegerOverflow=off
  Constant1 : Constant  Value=0.01
  Current Sensor1 : fl_lib/Electrical/Electrical Sensors/Current Sensor
  Current Sensor3 : fl_lib/Electrical/Electrical Sensors/Current Sensor
  Divide : Product  Inputs=*/
  Divide1 : Product  Inputs=*/
  Divide2 : Product  Inputs=**
  Electrical Reference3 : fl_lib/Electrical/Electrical Elements/Electrical Reference
  Electrical Reference4 : fl_lib/Electrical/Electrical Elements/Electrical Reference
  IC2 : InitialCondition
  Ideal Transformer with variable winding ratio : My_second_lib/Ideal Transformer with variable winding ratio  i1_specify=on  i1_priority=None  i1=0 A  i1_nominal_specify=off  i1_nominal_unit=A  i1_nominal_value=1  v1_specify=off  v1_priority=None  v1=3 V  v1_nominal_specify=off  v1_nominal_unit=V  v1_nominal_value=1  i2_specify=off  i2_priority=None  i2=0 A  i2_nominal_specify=off  i2_nominal_unit=A  i2_nominal_value=1  v2_specify=off  v2_priority=High  v2=5 V  v2_nominal_specify=off  v2_nominal_unit=V  v2_nominal_value=1
      settings: InternalSimscapePortConfiguration="{\"Bottom\":[],\"Left\":[{\"id\":\"p1\",\"label\":\"1+\",\"type\":\"foundation.electrical.electrical\"},{\"id\":\"n1\",\"label\":\"1-\",\"type\":\"foundation.electrical.electrical\"},{\"id\":\"n\",\"label\":\"Winding ratio input\",\"type\":\"input\"}],\"Right\":[{\"id\":\"p2\",\"label\":\"2+\",\"type\":\"foundation.electrical.electrical\"},{\"id\":\"n2\",\"label\":\"2-\",\"type\":\"foundation.electrical.electrical\"}],\"Top\":[]}"
  MATLAB Function2 : MATLAB Function  TreatAsAtomicUnit=on
  Math Function : Math  Operator=square
  PS-Simulink Converter{5..8} (4 alike) : nesl_utility/PS-Simulink Converter  PhysicalDomain=network_engine_domain  SubClassName=ps_output  LeftPortType=input  RightPortType=output  PseudoPeriodic=off  Frequencies=[]  VectorFormat=inherit  Unit=inherit  AffineConversion=off
  SPST Switch1 : ee_lib/Switches & Breakers/SPST Switch  R_closed=1e-6 Ohm  G_open=1e-6 S  Threshold=1 V  Width=0 V  model_dynamics=0  t_on=1e-3 s  t_off=1e-3 s  initial_vT=0 V
      settings: InternalSimscapePortConfiguration="{\"Bottom\":[],\"Left\":[{\"id\":\"vT\",\"label\":\"vT\",\"type\":\"input\"},{\"id\":\"p\",\"label\":\"\",\"type\":\"foundation.electrical.electrical\"}],\"Right\":[{\"id\":\"n\",\"label\":\"\",\"type\":\"foundation.electrical.electrical\"}],\"Top\":[]}"
  Scope : Scope  NumInputPorts=2
  Scope1 : Scope
  Simulink-PS Converter2 : nesl_utility/Simulink-PS Converter  PhysicalDomain=network_engine_domain  SubClassName=ps_input  LeftPortType=input  RightPortType=output  PseudoPeriodic=off  Frequencies=[]  NoiseDistribution=none  NoiseParameters=[]  Unit=V  AffineConversion=on  FilteringAndDerivatives=provide  SimscapeFilterOrder=1  InputFilterTimeConstant=0.001  UdotUserProvided=0
  Simulink-PS Converter3 : nesl_utility/Simulink-PS Converter  PhysicalDomain=network_engine_domain  SubClassName=ps_input  LeftPortType=input  RightPortType=output  PseudoPeriodic=off  Frequencies=[]  NoiseDistribution=none  NoiseParameters=[]  Unit=1  AffineConversion=off  FilteringAndDerivatives=provide  SimscapeFilterOrder=1  InputFilterTimeConstant=0.001  UdotUserProvided=0
  Simulink-PS Converter5 : nesl_utility/Simulink-PS Converter  PhysicalDomain=network_engine_domain  SubClassName=ps_input  LeftPortType=input  RightPortType=output  PseudoPeriodic=off  Frequencies=[]  NoiseDistribution=none  NoiseParameters=[]  Unit=1  AffineConversion=off  FilteringAndDerivatives=provide  SimscapeFilterOrder=1  InputFilterTimeConstant=0.001  UdotUserProvided=0
  Switch : Switch  Criteria=u2 > Threshold  Threshold=0.01  SaturateOnIntegerOverflow=off  InputSameDT=off
  Transport Delay : TransportDelay  DelayTime=1e-06
  Unit Delay1 : UnitDelay  SampleTime=-1  HasFrameUpgradeWarning=on
  V_s : Constant  Value=5
  Variable Resistor1 : fl_lib/Electrical/Electrical Elements/Variable Resistor  Rmin=0 Ohm  thermalEnable=false  thermal_mass=1 J/K  i_specify=off  i_priority=None  i=0 A  i_nominal_specify=off  i_nominal_unit=A  i_nominal_value=1  v_specify=off  v_priority=None  v=0 V  v_nominal_specify=off  v_nominal_unit=V  v_nominal_value=1  T_specify=off  T_priority=None  T=300 K  T_nominal_specify=off  T_nominal_unit=K  T_nominal_value=1
  Voltage Sensor2 : fl_lib/Electrical/Electrical Sensors/Voltage Sensor
  Voltage Sensor3 : fl_lib/Electrical/Electrical Sensors/Voltage Sensor
  + : PMIOPort  Side=Left
  - : PMIOPort  Port=2  Side=Left
  V_primario : Outport
  V_secondario : Outport  Port=2
  Power Output : Outport  Port=3
  wires:
  V_s/1 -> Divide/2
  PS-Simulink Converter5/1 -> MATLAB Function2/1(input), Abs/1, V_primario/1, Scope/1  "V_primario"
  Divide1/1 -> Simulink-PS Converter5/1
  Divide/1 -> IC2/1
  Abs/1 -> Divide/1
  Switch/1 -> Math Function/1, Simulink-PS Converter3/1
  PS-Simulink Converter8/1 -> Scope1/1  "I_primario"
  PS-Simulink Converter6/1 -> Divide2/2, V_secondario/1, Scope/2  "V_secondario"
  Transport Delay/1 -> Simulink-PS Converter2/1
  PS-Simulink Converter7/1 -> Divide2/1
  Math Function/1 -> Divide1/2
  Constant1/1 -> Switch/3
  IC2/1 -> Switch/2, Switch/1
  [R_te] -> Divide1/1
  Unit Delay1/1 -> MATLAB Function2/2(prevState)
  MATLAB Function2/1(y) -> Transport Delay/1, Unit Delay1/1
  Divide2/1 -> Power Output/1  "POwer output"
  connections:
  Voltage Sensor2/LConn1 -- SPST Switch1/LConn2 -- +/RConn1
  Electrical Reference3/LConn1 -- -/RConn1 -- Ideal Transformer with variable winding ratio/LConn2 -- Voltage Sensor2/RConn2
  Electrical Reference4/LConn1 -- Ideal Transformer with variable winding ratio/RConn2 -- Variable Resistor1/RConn1 -- Voltage Sensor3/RConn2
  Variable Resistor1/LConn2 -- Voltage Sensor3/LConn1 -- Current Sensor1/RConn2
  Voltage Sensor2/RConn1 -- PS-Simulink Converter5/LConn1
  Current Sensor3/RConn2 -- Ideal Transformer with variable winding ratio/LConn1
  Current Sensor1/RConn1 -- PS-Simulink Converter7/LConn1
  Simulink-PS Converter5/RConn1 -- Variable Resistor1/LConn1
  Simulink-PS Converter3/RConn1 -- Ideal Transformer with variable winding ratio/LConn3
  Simulink-PS Converter2/RConn1 -- SPST Switch1/LConn1
  SPST Switch1/RConn1 -- Current Sensor3/LConn1
  Ideal Transformer with variable winding ratio/RConn1 -- Current Sensor1/LConn1
  Current Sensor3/RConn1 -- PS-Simulink Converter8/LConn1
  Voltage Sensor3/RConn1 -- PS-Simulink Converter6/LConn1

== system pvt_tegs_vienna/Heat on PV ==
  Controlled Heat Flow Rate Source1 : fl_lib/Thermal/Thermal Sources/Controlled Heat Flow Rate Source
  Simulink-PS Converter9 : nesl_utility/Simulink-PS Converter  PhysicalDomain=network_engine_domain  SubClassName=ps_input  LeftPortType=input  RightPortType=output  PseudoPeriodic=off  Frequencies=[]  NoiseDistribution=none  NoiseParameters=[]  Unit=W  AffineConversion=off  FilteringAndDerivatives=provide  SimscapeFilterOrder=1  InputFilterTimeConstant=0.001  UdotUserProvided=0
  Thermal Reference2 : fl_lib/Thermal/Thermal Elements/Thermal Reference
  B : PMIOPort  Side=Left
  wires:
  [E] -> Simulink-PS Converter9/1
  connections:
  Simulink-PS Converter9/RConn1 -- Controlled Heat Flow Rate Source1/RConn1
  Thermal Reference2/LConn1 -- Controlled Heat Flow Rate Source1/RConn2
  Controlled Heat Flow Rate Source1/LConn1 -- B/RConn1

== system pvt_tegs_vienna/Heat on glass ==
  Controlled Heat Flow Rate Source : fl_lib/Thermal/Thermal Sources/Controlled Heat Flow Rate Source
  Simulink-PS Converter7 : nesl_utility/Simulink-PS Converter  PhysicalDomain=network_engine_domain  SubClassName=ps_input  LeftPortType=input  RightPortType=output  PseudoPeriodic=off  Frequencies=[]  NoiseDistribution=none  NoiseParameters=[]  Unit=W  AffineConversion=off  FilteringAndDerivatives=provide  SimscapeFilterOrder=1  InputFilterTimeConstant=0.001  UdotUserProvided=0
  Thermal Reference1 : fl_lib/Thermal/Thermal Elements/Thermal Reference
  B : PMIOPort  Side=Left
  wires:
  [D] -> Simulink-PS Converter7/1
  connections:
  Simulink-PS Converter7/RConn1 -- Controlled Heat Flow Rate Source/RConn1
  Controlled Heat Flow Rate Source/RConn2 -- Thermal Reference1/LConn1
  Controlled Heat Flow Rate Source/LConn1 -- B/RConn1

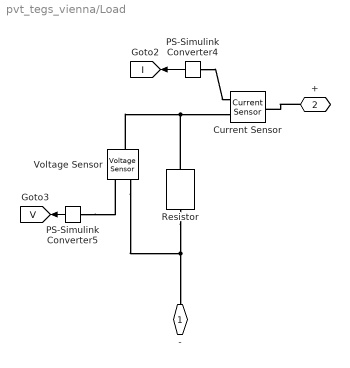
== system pvt_tegs_vienna/Load ==
  Current Sensor : fl_lib/Electrical/Electrical Sensors/Current Sensor
  PS-Simulink Converter4 : nesl_utility/PS-Simulink Converter  PhysicalDomain=network_engine_domain  SubClassName=ps_output  LeftPortType=input  RightPortType=output  PseudoPeriodic=off  Frequencies=[]  VectorFormat=1-D array  Unit=1  AffineConversion=off
  PS-Simulink Converter5 : nesl_utility/PS-Simulink Converter  PhysicalDomain=network_engine_domain  SubClassName=ps_output  LeftPortType=input  RightPortType=output  PseudoPeriodic=off  Frequencies=[]  VectorFormat=1-D array  Unit=1  AffineConversion=off
  Resistor : fl_lib/Electrical/Electrical Elements/Resistor  R=load.R Ohm  i_specify=off  i_priority=None  i=0 A  i_nominal_specify=off  i_nominal_unit=A  i_nominal_value=1  v_specify=off  v_priority=None  v=0 V  v_nominal_specify=off  v_nominal_unit=V  v_nominal_value=1
  Voltage Sensor : fl_lib/Electrical/Electrical Sensors/Voltage Sensor
  - : PMIOPort  Side=Left
  + : PMIOPort  Port=2  Side=Right
  tag scope: I=global, V=global
  wires:
  PS-Simulink Converter4/1 -> [I]
  PS-Simulink Converter5/1 -> [V]
  connections:
  +/RConn1 -- Current Sensor/LConn1
  PS-Simulink Converter5/LConn1 -- Voltage Sensor/RConn1
  PS-Simulink Converter4/LConn1 -- Current Sensor/RConn1
  Voltage Sensor/LConn1 -- Resistor/LConn1 -- Current Sensor/RConn2
  Resistor/RConn1 -- Voltage Sensor/RConn2 -- -/RConn1

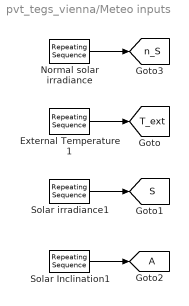
== system pvt_tegs_vienna/Meteo inputs ==
  " Solar Inclination1" : simulink/Sources/Repeating Sequence  rep_seq_t=time  rep_seq_y=Inclination.(month)
  External Temperature1 : simulink/Sources/Repeating Sequence  rep_seq_t=time  rep_seq_y=T_ext.(month)
  Goto2 : Goto  TagVisibility=global
  Normal solar irradiance : simulink/Sources/Repeating Sequence  rep_seq_t=time  rep_seq_y=Irradiance_si.(month)
  Solar irradiance1 : simulink/Sources/Repeating Sequence  rep_seq_t=time  rep_seq_y=Irradiance_ts.(month)
  tag scope: S=global, T_ext=global, n_S=global
  wires:
  External Temperature1/1 -> [T_ext]
  " Solar Inclination1"/1 -> Goto2/1
  Solar irradiance1/1 -> [S]
  Normal solar irradiance/1 -> [n_S]

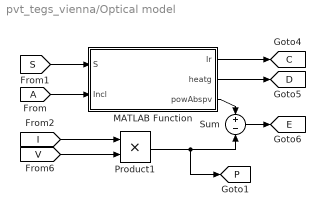
== system pvt_tegs_vienna/Optical model ==
  From : From  TagVisibility=global
  MATLAB Function : MATLAB Function  TreatAsAtomicUnit=on
  Product1 : Product
  Sum : Sum  Inputs=+-
  tag scope: C=global, D=global, E=global, P=global
  wires:
  MATLAB Function/1(Ir) -> [C]
  Sum/1 -> [E]
  MATLAB Function/2(heatg) -> [D]
  MATLAB Function/3(powAbspv) -> Sum/1
  Product1/1 -> Sum/2, [P]
  [I] -> Product1/1
  [V] -> Product1/2
  From/1 -> MATLAB Function/2(Incl)
  [S] -> MATLAB Function/1(S)

== system pvt_tegs_vienna/Pump ==
  Controlled Mass Flow Rate Source (TL)5 : fl_lib/Thermal Liquid/Sources/Flow Rate Source (TL)  source_type=foundation.enum.constant_controlled.controlled  flow_type=foundation.enum.mass_volumetric_flow.mass  mass_flow=0 kg/s  volumetric_flow=0 m^3/s  power_spec=foundation.enum.power_spec.isentropic  area=0.01 m^2
  Simulink-PS Converter10 : nesl_utility/Simulink-PS Converter  PhysicalDomain=network_engine_domain  SubClassName=ps_input  LeftPortType=input  RightPortType=output  PseudoPeriodic=off  Frequencies=[]  NoiseDistribution=none  NoiseParameters=[]  Unit=kg/s  AffineConversion=off  FilteringAndDerivatives=provide  SimscapeFilterOrder=1  InputFilterTimeConstant=0.001  UdotUserProvided=0
  B : PMIOPort  Side=Right
  A : PMIOPort  Port=2  Side=Left
  wires:
  [J] -> Simulink-PS Converter10/1
  connections:
  Controlled Mass Flow Rate Source (TL)5/LConn1 -- A/RConn1
  Simulink-PS Converter10/RConn1 -- Controlled Mass Flow Rate Source (TL)5/LConn2
  B/RConn1 -- Controlled Mass Flow Rate Source (TL)5/RConn1

== system pvt_tegs_vienna/Pump flow inputs ==
  internal_flow : simulink/Sources/Repeating Sequence  rep_seq_t="[0, 3600*6, 3600*6+0.1,  3600*22, 3600*22+0.1, 3600*24]"  rep_seq_y=pumps.mdot_int*[1,1,1,1,1,1]
  tag scope: J=global
  wires:
  internal_flow/1 -> [J]
